simulink model "exp12"  (R2023a)
settings: Solver=VariableStepAuto  StartTime=0.0  StopTime=0.08  RelTol=1e-3
libraries: spsSeriesRLCBranchLib x4, spsCurrentMeasurementLib x2, spsIGBTDiodeLib x2, spsDCVoltageSourceLib x1, spsMultimeterLib x1, spsVoltageMeasurementLib x1, sps_lib x1
settings Model: Creator=Asus  LastModifiedBy=pc
settings RTWCC: GPUComputeCapability=5.0

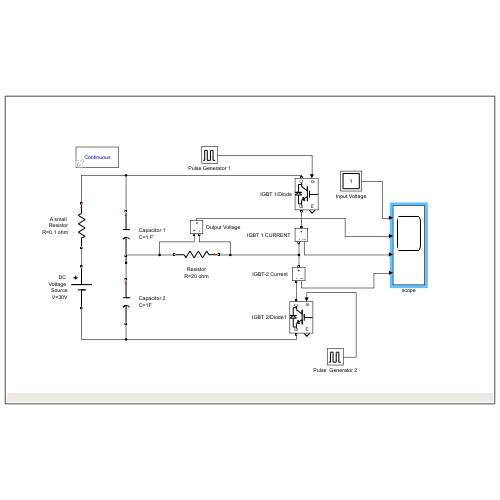
[thumbnail: Simulink's stored preview of the top-level diagram]
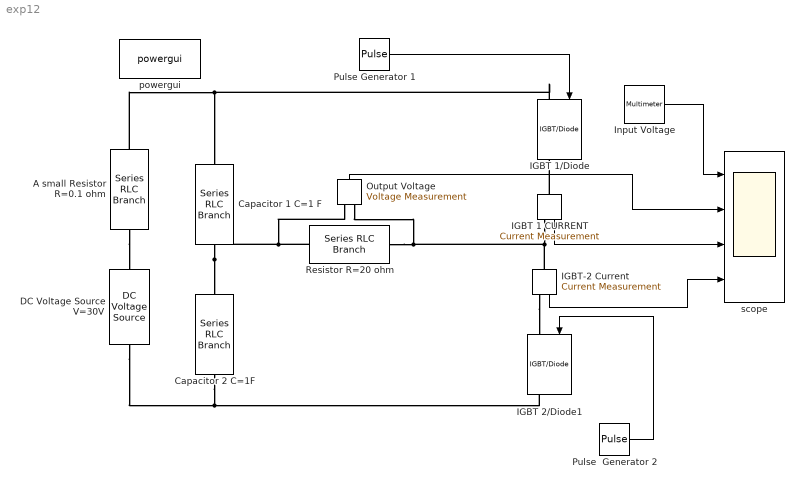
== system exp12 ==
  A small Resistor R=0.1 ohm : spsSeriesRLCBranchLib/Series RLC Branch  LConnTagsString=__new0  RConnTagsString=__new0  BranchType=R  Resistance=0.1  Inductance=1e-3  SetiL0=off  InitialCurrent=0  Capacitance=1e-6  Setx0=off  InitialVoltage=0  Measurements=None
  Capacitor 1 C=1 F : spsSeriesRLCBranchLib/Series RLC Branch  LConnTagsString=__new0  RConnTagsString=__new0  BranchType=C  Resistance=1  Inductance=1e-3  SetiL0=off  InitialCurrent=0  Capacitance=1  Setx0=off  InitialVoltage=0  Measurements=None
  Capacitor 2 C=1F : spsSeriesRLCBranchLib/Series RLC Branch  LConnTagsString=__new0  RConnTagsString=__new0  BranchType=C  Resistance=1  Inductance=1e-3  SetiL0=off  InitialCurrent=0  Capacitance=1  Setx0=off  InitialVoltage=0  Measurements=None
  DC Voltage Source V=30V : spsDCVoltageSourceLib/DC Voltage Source  Amplitude=30  Measurements=Voltage
  "IGBT 1 CURRENT " : spsCurrentMeasurementLib/Current Measurement  PhasorSimulation=off  OutputType=Complex  PSBequivalent=0
  IGBT 1/Diode : spsIGBTDiodeLib/IGBT//Diode  Ron=1e-3  Rs=1e5  Cs=inf  Measurements=on
  IGBT 2/Diode1 : spsIGBTDiodeLib/IGBT//Diode  Ron=1e-3  Rs=1e5  Cs=inf  Measurements=on
  "IGBT-2 Current " : spsCurrentMeasurementLib/Current Measurement  PhasorSimulation=off  OutputType=Complex  PSBequivalent=0
  Input Voltage : spsMultimeterLib/Multimeter  L=1  sel=1  yselected={}  Gain=1  OutputType=Complex  PlotAtSimulationStop=off  PhasorSimulation=off
  Output Voltage : spsVoltageMeasurementLib/Voltage Measurement  PhasorSimulation=off  OutputType=Complex  PSBequivalent=0
  Pulse  Generator 2 : DiscretePulseGenerator  PulseType=Time based  Period=0.02  PulseWidth=50  PhaseDelay=(180/360)*0.02
  Pulse Generator 1 : DiscretePulseGenerator  PulseType=Time based  Period=0.02  PulseWidth=50  PhaseDelay=(0/360)*0.02
  Resistor R=20 ohm : spsSeriesRLCBranchLib/Series RLC Branch  LConnTagsString=__new0  RConnTagsString=__new0  BranchType=R  Resistance=20  Inductance=1e-3  SetiL0=off  InitialCurrent=0  Capacitance=1e-6  Setx0=off  InitialVoltage=0  Measurements=None
  powergui : sps_lib/powergui  Priority=1  SimulationMode=Continuous  SampleTime=50e-6  frequency=60  Iterations=50  frequencyindice=0  Pbase=100e6  ErrMax=1e-4  UnitsV=kV  UnitsW=MW  buscounter=0  FunctionMessages=off  echomessages=off  EnableUseOfTLC=off  CurrentSourceSwitches=off  DisableSnubberDevices=off  DisableRonSwitches=off  DisableVfSwitches=off  DisplayEquations=off  AutomaticDiscreteSolvers=off  SolverType=Tustin/Backward Euler (TBE)  Interpol=off  ExternalGateDelay=off  methode=off  Ts=100  x0status=blocks  SPID=on  SwTol=0  HookPort=off  NonlinearTolerance=1e-4  nMaxIteration=100  ContinueOnMaxIteration=off  RestoreLinks=warning  ResistiveCurrentMeasurement=off  Frange=[0:2:500]  Ylog=off  Xlog=on  ShowGrid=off  save=off  variable=ZData  structure=0  ZoomFFT=off  StartTime=0.0  cycles=1  DisplayStyle=1  fundamental=60  FreqAxis=off  MaxFrequency=1000  frequencyindicesteady=1  RmsSteady=1  display=off
  scope : Scope  NumInputPorts=4
  wires:
  Pulse  Generator 2/1 -> IGBT 2/Diode1/1
  Pulse Generator 1/1 -> IGBT 1/Diode/1
  Output Voltage/1 -> scope/2
  "IGBT 1 CURRENT "/1 -> scope/3
  "IGBT-2 Current "/1 -> scope/4
  Input Voltage/1 -> scope/1
  connections:
  A small Resistor R=0.1 ohm/RConn1 -- DC Voltage Source V=30V/RConn1
  A small Resistor R=0.1 ohm/LConn1 -- IGBT 1/Diode/LConn1 -- Capacitor 1 C=1 F/LConn1
  Capacitor 1 C=1 F/RConn1 -- Resistor R=20 ohm/RConn1 -- Output Voltage/LConn1 -- Capacitor 2 C=1F/LConn1
  Resistor R=20 ohm/LConn1 -- "IGBT-2 Current "/LConn1 -- "IGBT 1 CURRENT "/RConn1 -- Output Voltage/LConn2
  DC Voltage Source V=30V/LConn1 -- Capacitor 2 C=1F/RConn1 -- IGBT 2/Diode1/RConn1
  "IGBT 1 CURRENT "/LConn1 -- IGBT 1/Diode/RConn1
  "IGBT-2 Current "/RConn1 -- IGBT 2/Diode1/LConn1
